simulink library "GT"  (R2024a)
settings: Solver=VariableStepAuto  StartTime=0.0  StopTime=10.0  RelTol=1e-3
undefined symbols (not defined in the file): aero, cb, Earth, geo, initcond, WGS84
libraries: simulink_extras x10, aerolibactuator x5, shared6dof x1, AeroLoads x1, aerolibtransform2 x1, simulink x1, PropLoads x1
settings Model: Creator=igmso  LastModifiedBy=igmso

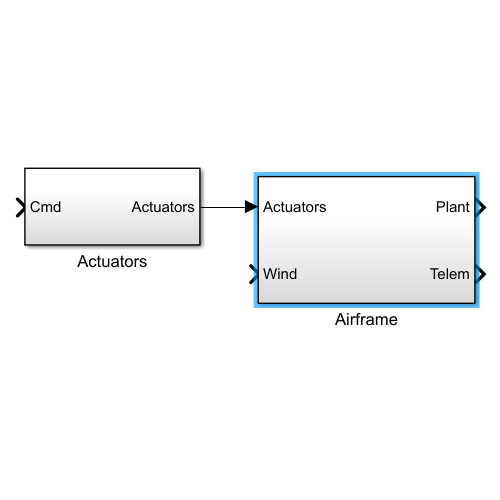
[thumbnail: Simulink's stored preview of the top-level diagram]
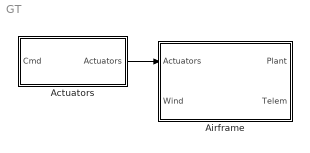
== system GT ==
  Actuators : Subsystem
  Airframe : Subsystem
  wires:
  Actuators/1(Actuators) -> Airframe/1(Actuators)

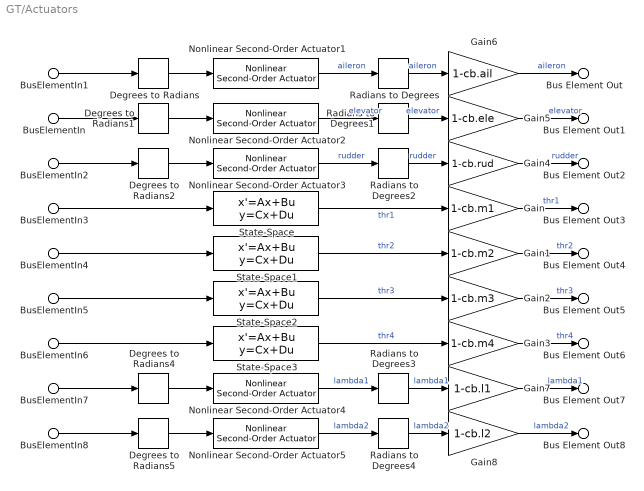
== system GT/Actuators ==
  BusElementIn1 : Inport  PortName=Cmd  Element=aileron
  BusElementIn : Inport  PortName=Cmd  Element=elevator
  BusElementIn2 : Inport  PortName=Cmd  Element=rudder
  BusElementIn3 : Inport  PortName=Cmd  Element=thr1
  BusElementIn4 : Inport  PortName=Cmd  Element=thr2
  BusElementIn5 : Inport  PortName=Cmd  Element=thr3
  BusElementIn6 : Inport  PortName=Cmd  Element=thr4
  BusElementIn7 : Inport  PortName=Cmd  Element=lambda1
  BusElementIn8 : Inport  PortName=Cmd  Element=lambda2
  Degrees to Radians{,1..2,4..5} (5 alike) : simulink_extras/Transformations/Degrees to Radians
  Gain : Gain  Gain=1-cb.m1
  Gain1 : Gain  Gain=1-cb.m2
  Gain2 : Gain  Gain=1-cb.m3
  Gain3 : Gain  Gain=1-cb.m4
  Gain4 : Gain  Gain=1-cb.rud
  Gain5 : Gain  Gain=1-cb.ele
  Gain6 : Gain  Gain=1-cb.ail
  Gain7 : Gain  Gain=1-cb.l1
  Gain8 : Gain  Gain=1-cb.l2
  Nonlinear Second-Order Actuator1 : aerolibactuator/Nonlinear Second-Order Actuator  wn_fin=60  z_fin=0.7  fin_max=deg2rad(15)  fin_min=-deg2rad(15)  fin_maxrate=6.16  fin_act_0=deg2rad(initcond.aileron)  fin_act_vel=0
  Nonlinear Second-Order Actuator2 : aerolibactuator/Nonlinear Second-Order Actuator  wn_fin=60  z_fin=0.7  fin_max=deg2rad(30)  fin_min=-deg2rad(30)  fin_maxrate=6.16  fin_act_0=deg2rad(initcond.elevator)  fin_act_vel=0
  Nonlinear Second-Order Actuator3 : aerolibactuator/Nonlinear Second-Order Actuator  wn_fin=60  z_fin=0.7  fin_max=deg2rad(30)  fin_min=-deg2rad(30)  fin_maxrate=6.16  fin_act_0=deg2rad(initcond.rudder)  fin_act_vel=0
  Nonlinear Second-Order Actuator4 : aerolibactuator/Nonlinear Second-Order Actuator  wn_fin=60  z_fin=0.7  fin_max=deg2rad(90)  fin_min=0  fin_maxrate=6.16  fin_act_0=deg2rad(initcond.lambda1)  fin_act_vel=0
  Nonlinear Second-Order Actuator5 : aerolibactuator/Nonlinear Second-Order Actuator  wn_fin=60  z_fin=0.7  fin_max=deg2rad(90)  fin_min=0  fin_maxrate=6.16  fin_act_0=deg2rad(initcond.lambda2)  fin_act_vel=0
  Radians to Degrees{,1..4} (5 alike) : simulink_extras/Transformations/Radians to Degrees
  State-Space : StateSpace  A=-10  B=10  D=0  InitialCondition=initcond.thr1
  State-Space1 : StateSpace  A=-10  B=10  D=0  InitialCondition=initcond.thr2
  State-Space2 : StateSpace  A=-10  B=10  D=0  InitialCondition=initcond.thr3
  State-Space3 : StateSpace  A=-10  B=10  D=0  InitialCondition=initcond.thr4
  Bus Element Out : Outport  PortName=Actuators  Element=aileron
  Bus Element Out1 : Outport  PortName=Actuators  Element=elevator
  Bus Element Out2 : Outport  PortName=Actuators  Element=rudder
  Bus Element Out3 : Outport  PortName=Actuators  Element=thr1
  Bus Element Out4 : Outport  PortName=Actuators  Element=thr2
  Bus Element Out5 : Outport  PortName=Actuators  Element=thr3
  Bus Element Out6 : Outport  PortName=Actuators  Element=thr4
  Bus Element Out7 : Outport  PortName=Actuators  Element=lambda1
  Bus Element Out8 : Outport  PortName=Actuators  Element=lambda2
  wires:
  BusElementIn3/1 -> State-Space/1
  BusElementIn4/1 -> State-Space1/1
  BusElementIn5/1 -> State-Space2/1
  BusElementIn6/1 -> State-Space3/1
  BusElementIn7/1 -> Degrees to Radians4/1
  BusElementIn8/1 -> Degrees to Radians5/1
  BusElementIn2/1 -> Degrees to Radians2/1
  BusElementIn/1 -> Degrees to Radians1/1
  BusElementIn1/1 -> Degrees to Radians/1
  Radians to Degrees4/1 -> Gain8/1  "lambda2"
  Radians to Degrees3/1 -> Gain7/1  "lambda1"
  State-Space3/1 -> Gain3/1  "thr4"
  State-Space2/1 -> Gain2/1  "thr3"
  State-Space1/1 -> Gain1/1  "thr2"
  State-Space/1 -> Gain/1  "thr1"
  Radians to Degrees2/1 -> Gain4/1  "rudder"
  Radians to Degrees1/1 -> Gain5/1  "elevator"
  Radians to Degrees/1 -> Gain6/1  "aileron"
  Nonlinear Second-Order Actuator3/1 -> Radians to Degrees2/1  "rudder"
  Nonlinear Second-Order Actuator2/1 -> Radians to Degrees1/1  "elevator"
  Nonlinear Second-Order Actuator1/1 -> Radians to Degrees/1  "aileron"
  Nonlinear Second-Order Actuator4/1 -> Radians to Degrees3/1  "lambda1"
  Nonlinear Second-Order Actuator5/1 -> Radians to Degrees4/1  "lambda2"
  Degrees to Radians5/1 -> Nonlinear Second-Order Actuator5/1
  Degrees to Radians4/1 -> Nonlinear Second-Order Actuator4/1
  Degrees to Radians2/1 -> Nonlinear Second-Order Actuator3/1
  Degrees to Radians1/1 -> Nonlinear Second-Order Actuator2/1
  Degrees to Radians/1 -> Nonlinear Second-Order Actuator1/1
  Gain7/1 -> Bus Element Out7/1  "lambda1"
  Gain1/1 -> Bus Element Out4/1  "thr2"
  Gain8/1 -> Bus Element Out8/1  "lambda2"
  Gain/1 -> Bus Element Out3/1  "thr1"
  Gain6/1 -> Bus Element Out/1  "aileron"
  Gain3/1 -> Bus Element Out6/1  "thr4"
  Gain4/1 -> Bus Element Out2/1  "rudder"
  Gain2/1 -> Bus Element Out5/1  "thr3"
  Gain5/1 -> Bus Element Out1/1  "elevator"

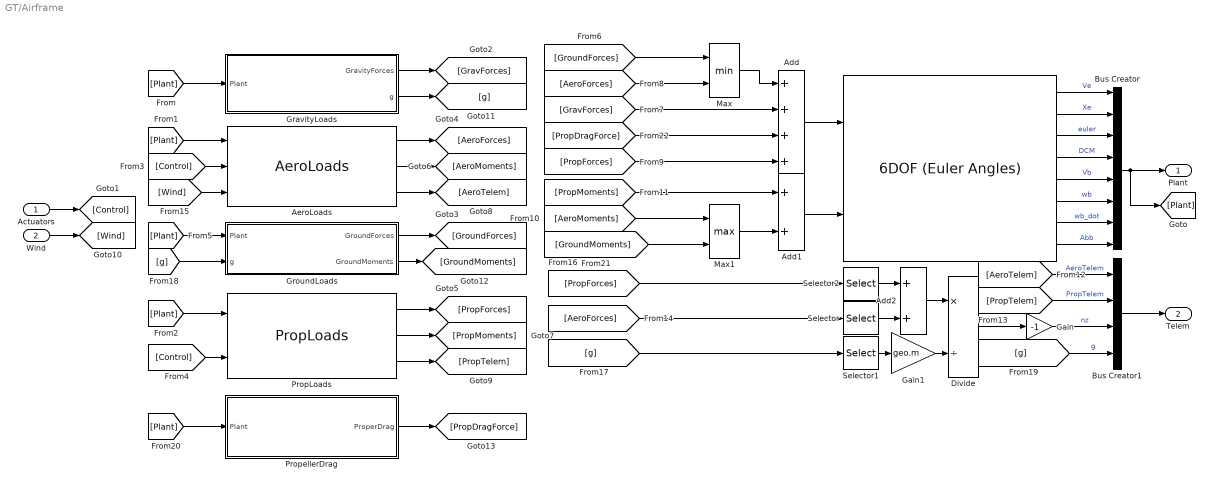
== system GT/Airframe ==
  Actuators : Inport
  Wind : Inport  Port=2
  " " : shared6dof/6DOF (Euler Angles)  units=Metric (MKS)  mtype=Fixed  rep=Euler Angles  xme_0=initcond.Xe0  Vm_0=initcond.Vb0  eul_0=initcond.euler0  pm_0=initcond.wb0  mass_0=geo.m  mass_e=0.5  mass_f=2.0  inertia=geo.Jbb  inertia_e=eye(3)  inertia_f=2*eye(3)  k_quat=1.0  vre_flag=on  abi_flag=off  aMode=0  xme_statename={'Xe', 'Ye', 'Ze'}  Vm_statename={'u', 'v', 'w'}  eul_statename={'phi', 'theta', 'psi'}  quat_statename=''  pm_statename={'p', 'q', 'r'}  mass_statename=''
      settings: LibrarySourceBlock=aerolib6dof2/6DOF (Quaternion)
  Add : Sum  Inputs=4
  Add1 : Sum
  Add2 : Sum
  AeroLoads : AeroLoads/AeroLoads  SystemSampleTime=-1  VariantActivationTime=update diagram  AllowFlexibleInterface=on  Latency=0  AutoFrameSizeCalculation=off
  Bus Creator1 : BusCreator  Inputs=4
  Bus Creator : BusCreator  Inputs=8
  Divide : Product  Inputs=*/
  Gain : Gain  Gain=-1
  Gain1 : Gain  Gain=geo.m
  GravityLoads : Subsystem
  GroundLoads : Subsystem
  Max : MinMax  Inputs=2
  Max1 : MinMax  Function=max  Inputs=2
  PropLoads : PropLoads/PropLoads  SystemSampleTime=-1  VariantActivationTime=update diagram  AllowFlexibleInterface=on  Latency=0  AutoFrameSizeCalculation=off
  PropellerDrag : Subsystem
  Selector : Selector  InputPortWidth=3  IndexOptions=Index vector (dialog)  Indices=3  OutputSizes=1
  Selector1 : Selector  InputPortWidth=3  IndexOptions=Index vector (dialog)  Indices=3  OutputSizes=1
  Selector2 : Selector  InputPortWidth=3  IndexOptions=Index vector (dialog)  Indices=3  OutputSizes=1
  Plant : Outport
  Telem : Outport  Port=2
  wires:
  [AeroMoments] -> Max1/1
  Max1/1 -> Add1/2
  [GravForces] -> Add/2
  [PropForces] -> Add/4
  Max/1 -> Add/1
  [GroundMoments] -> Max1/2
  GroundLoads/2(GroundMoments) -> [GroundMoments]
  [g] -> Bus Creator1/4  "g"
  [g] -> GroundLoads/2(g)
  Gain/1 -> Bus Creator1/3  "nz"
  " "/8 -> Bus Creator/8  "Abb"
  Add2/1 -> Divide/1
  Selector2/1 -> Add2/1
  [PropForces] -> Selector2/1
  Gain1/1 -> Divide/2
  Selector1/1 -> Gain1/1
  [g] -> Selector1/1
  GravityLoads/2(g) -> [g]
  [Wind] -> AeroLoads/3
  [AeroForces] -> Max/2
  " "/1 -> Bus Creator/1  "Ve"
  " "/2 -> Bus Creator/2  "Xe"
  [PropMoments] -> Add1/1
  AeroLoads/2 -> [AeroMoments]
  [Control] -> PropLoads/2
  Actuators/1 -> [Control]
  " "/4 -> Bus Creator/4  "DCM"
  [GroundForces] -> Max/1
  [Control] -> AeroLoads/2
  Add/1 -> " "/1
  Bus Creator/1 -> [Plant], Plant/1
  PropLoads/3 -> [PropTelem]
  " "/3 -> Bus Creator/3  "euler"
  Add1/1 -> " "/2
  " "/7 -> Bus Creator/7  "wb_dot"
  " "/6 -> Bus Creator/6  "wb"
  GravityLoads/1(GravityForces) -> [GravForces]
  PropLoads/1 -> [PropForces]
  " "/5 -> Bus Creator/5  "Vb"
  [Plant] -> GroundLoads/1(Plant)
  GroundLoads/1(GroundForces) -> [GroundForces]
  AeroLoads/1 -> [AeroForces]
  [Plant] -> PropLoads/1
  PropLoads/2 -> [PropMoments]
  [Plant] -> AeroLoads/1
  [Plant] -> GravityLoads/1(Plant)
  AeroLoads/3 -> [AeroTelem]
  [AeroTelem] -> Bus Creator1/1  "AeroTelem"
  [PropTelem] -> Bus Creator1/2  "PropTelem"
  Bus Creator1/1 -> Telem/1
  [AeroForces] -> Selector/1
  Selector/1 -> Add2/2
  Divide/1 -> Gain/1
  Wind/1 -> [Wind]
  [Plant] -> PropellerDrag/1(Plant)
  PropellerDrag/1(ProperDrag) -> [PropDragForce]
  [PropDragForce] -> Add/3

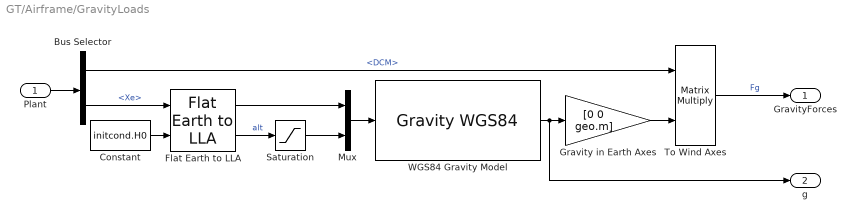
== system GT/Airframe/GravityLoads ==
  Plant : Inport
  Bus Selector : BusSelector  OutputSignals=DCM,Xe
  Constant : Constant  Value=initcond.H0  SampleTime=-1
  Flat Earth to LLA : aerolibtransform2/Flat Earth to LLA  units=Metric (MKS)  ptype=Earth (WGS84)  F=1/298.257223563  R=6378137  refPosPort=off  LL0=[-23.2296 -45.8614].'  psi=150
  Gravity in Earth Axes : Gain  Gain=[0 0 geo.m]  SaturateOnIntegerOverflow=on  OutDataTypeStr=Inherit: Same as input  ParamDataTypeStr=Inherit: Same as input
  Mux : Mux  Inputs=2
  Saturation : Saturate  UpperLimit=20e3  LowerLimit=0
  To Wind Axes : Product  Multiplication=Matrix(*)  InputSameDT=on  SaturateOnIntegerOverflow=on  OutDataTypeStr=Inherit: Same as first input
  "WGS84 Gravity Model  " : GravityWGS84
  GravityForces : Outport
  g : Outport  Port=2
  wires:
  Saturation/1 -> Mux/2
  Mux/1 -> "WGS84 Gravity Model  "/1
  Bus Selector/1 -> To Wind Axes/1  "<DCM>"
  Flat Earth to LLA/2 -> Saturation/1  "alt"
  Gravity in Earth Axes/1 -> To Wind Axes/2
  Constant/1 -> Flat Earth to LLA/2
  "WGS84 Gravity Model  "/1 -> Gravity in Earth Axes/1, g/1
  Flat Earth to LLA/1 -> Mux/1
  Bus Selector/2 -> Flat Earth to LLA/1  "<Xe>"
  To Wind Axes/1 -> GravityForces/1  "Fg"
  Plant/1 -> Bus Selector/1

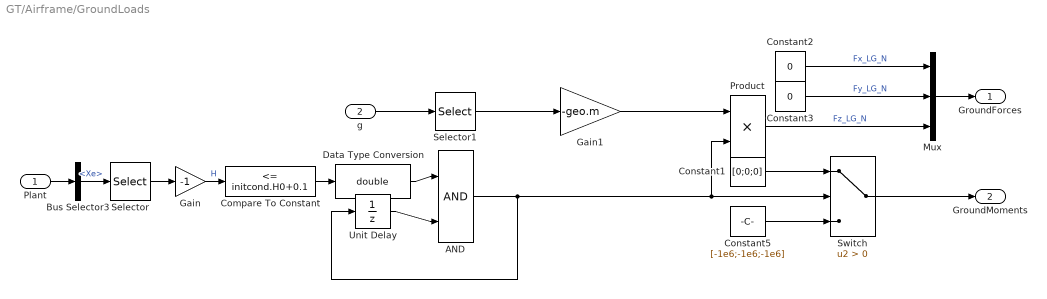
== system GT/Airframe/GroundLoads ==
  Plant : Inport
  g : Inport  Port=2
  AND : Logic  IconShape=distinctive  AllPortsSameDT=off  OutDataTypeStr=boolean
  Bus Selector3 : BusSelector  OutputSignals=Xe
  Compare To Constant : simulink/Logic and Bit Operations/Compare To Constant  relop=<=  const=initcond.H0+0.1  OutDataTypeStr=boolean
  Constant1 : Constant  Value=[0;0;0]  SampleTime=-1
  Constant2 : Constant  Value=0  SampleTime=-1
  Constant3 : Constant  Value=0  SampleTime=-1
  Constant5 : Constant  Value=[-1e6;-1e6;-1e6]  SampleTime=-1
  Data Type Conversion : DataTypeConversion  OutDataTypeStr=double  SaturateOnIntegerOverflow=off  RndMeth=Floor
  Gain : Gain  Gain=-1
  Gain1 : Gain  Gain=-geo.m
  Mux : Mux  Inputs=3
  Product : Product
  Selector : Selector  InputPortWidth=3  IndexOptions=Index vector (dialog)  Indices=3  OutputSizes=1
  Selector1 : Selector  InputPortWidth=3  IndexOptions=Index vector (dialog)  Indices=3  OutputSizes=1
  Switch : Switch  Criteria=u2 > Threshold  SaturateOnIntegerOverflow=off  InputSameDT=off
  Unit Delay : UnitDelay  InitialCondition=1  SampleTime=-1  HasFrameUpgradeWarning=on
  GroundForces : Outport
  GroundMoments : Outport  Port=2
  wires:
  Unit Delay/1 -> AND/2
  Data Type Conversion/1 -> AND/1
  Constant5/1 -> Switch/3
  Constant1/1 -> Switch/1
  Switch/1 -> GroundMoments/1
  Selector1/1 -> Gain1/1
  g/1 -> Selector1/1
  Bus Selector3/1 -> Selector/1  "<Xe>"
  Gain1/1 -> Product/1
  Compare To Constant/1 -> Data Type Conversion/1
  AND/1 -> Switch/2, Product/2, Unit Delay/1
  Plant/1 -> Bus Selector3/1
  Gain/1 -> Compare To Constant/1  "H"
  Constant2/1 -> Mux/1  "Fx_LG_N"
  Constant3/1 -> Mux/2  "Fy_LG_N"
  Product/1 -> Mux/3  "Fz_LG_N"
  Mux/1 -> GroundForces/1
  Selector/1 -> Gain/1

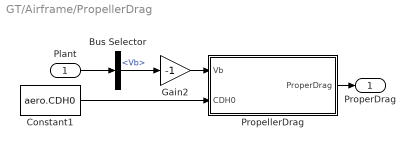
== system GT/Airframe/PropellerDrag ==
  Plant : Inport
  Bus Selector : BusSelector  OutputSignals=Vb
  Constant1 : Constant  Value=aero.CDH0  SampleTime=-1
  Gain2 : Gain  Gain=-1
  PropellerDrag : MATLAB Function  TreatAsAtomicUnit=on
  ProperDrag : Outport
  wires:
  Bus Selector/1 -> Gain2/1  "<Vb>"
  Plant/1 -> Bus Selector/1
  Constant1/1 -> PropellerDrag/2(CDH0)
  PropellerDrag/1(ProperDrag) -> ProperDrag/1
  Gain2/1 -> PropellerDrag/1(Vb)

== matlab function GT/Airframe/PropellerDrag/PropellerDrag ==
  data: Vb input; ProperDrag output; CDH0 input
function ProperDrag = fcn(Vb, CDH0)

ProperDrag = CDH0 * norm(Vb) * Vb;

end
